simulink library "fast_library"  (Simulink 8.1)
settings: Solver=ode45  StartTime=0.0  StopTime=10.0  RelTol=1e-3
libraries: xbsIndex_r4 x439, casper_library_misc x3, xps_library x2
(part 2 of 3)

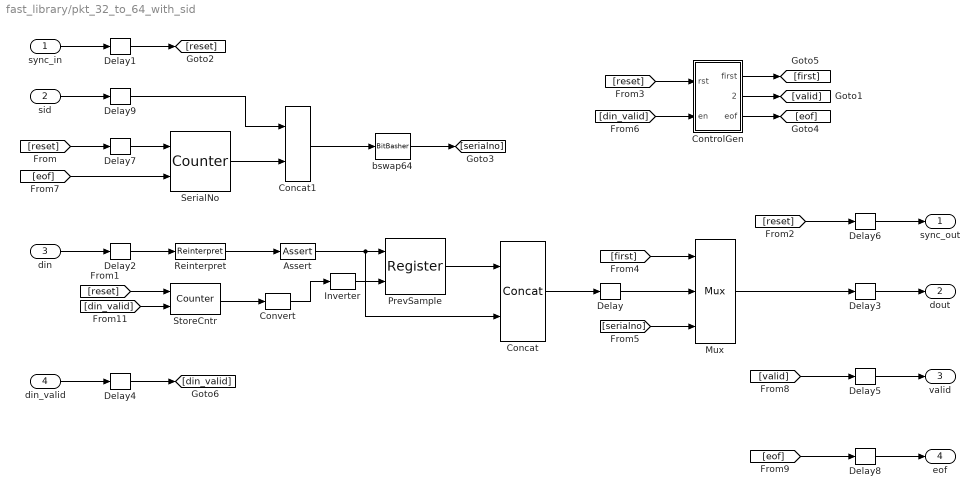
== system fast_library/pkt_32_to_64_with_sid ==
  sync_in : Inport
  sid : Inport  Port=2
  din : Inport  Port=3
  din_valid : Inport  Port=4
  Assert : xbsIndex_r4/Assert  assert_type=on  type_source=Explicitly  gui_display_data_type=Fixed-point  arith_type=Unsigned  n_bits=32  bin_pt=0  preci_type=Single  exp_width=8  frac_width=24  assert_rate=off  rate_source=Explicitly  period=1  output_port=on  block_type=assert
  Concat : xbsIndex_r4/Concat  num_inputs=2  dbl_ovrd=off  block_type=concat
  Concat1 : xbsIndex_r4/Concat  num_inputs=2  dbl_ovrd=off  block_type=concat
  ControlGen : Subsystem
  Convert : xbsIndex_r4/Convert  gui_display_data_type=Boolean  arith_type=Boolean  n_bits=16  bin_pt=14  float_type=Single  exp_bits=8  fraction_bits=24  quantization=Truncate  overflow=Wrap  en=off  latency=0  dbl_ovrd=off  pipeline=off  block_type=convert
  Delay{,1..5,7..9} (9 alike) : xbsIndex_r4/Delay  rst=off  infoeditControl=Selection of Reset will increase slice count due to use of real FFs and instead of SRLs  en=off  latency=1  dbl_ovrd=off  reg_retiming=off  block_type=delay
  Delay6 : xbsIndex_r4/Delay  rst=off  infoeditControl=Selection of Reset will increase slice count due to use of real FFs and instead of SRLs  en=off  latency=2  dbl_ovrd=off  reg_retiming=off  block_type=delay
  Inverter : xbsIndex_r4/Inverter  en=off  latency=0  dbl_ovrd=off  block_type=inv
  Mux : xbsIndex_r4/Mux  inputs=2  en=off  latency=0  precision=Full  arith_type=Unsigned  n_bits=16  bin_pt=14  quantization=Truncate  overflow=Wrap  dbl_ovrd=off  block_type=mux
  PrevSample : xbsIndex_r4/Register  init=0  rst=off  en=on  dbl_ovrd=off  block_type=register
  Reinterpret : xbsIndex_r4/Reinterpret  force_arith_type=on  arith_type=Unsigned  force_bin_pt=on  bin_pt=0  block_type=reinterpret
  SerialNo : xbsIndex_r4/Counter  cnt_type=Free Running  cnt_to=Inf  operation=Up  start_count=0  cnt_by_val=1  arith_type=Unsigned  n_bits=56  bin_pt=0  load_pin=off  rst=on  en=on  explicit_period=on  period=1  dbl_ovrd=off  use_behavioral_HDL=on  implementation=Fabric  block_type=counter
  StoreCntr : xbsIndex_r4/Counter  cnt_type=Free Running  cnt_to=Inf  operation=Up  start_count=0  cnt_by_val=1  arith_type=Unsigned  n_bits=1  bin_pt=0  load_pin=off  rst=on  en=on  explicit_period=on  period=1  dbl_ovrd=off  use_behavioral_HDL=off  implementation=Fabric  block_type=counter
  bswap64 : xbsIndex_r4/BitBasher  bitexpr=|  display_expr=off  sr_1=1  arith_type1=Unsigned  bin_pt1=0  sr_2=2  arith_type2=Unsigned  bin_pt2=0  sr_3=3  arith_type3=Unsigned  bin_pt3=0  sr_4=4  arith_type4=Unsigned  bin_pt4=0  dbl_ovrd=off  block_type=bitbasher
      | <!DOCTYPE HTML PUBLIC "-//W3C//DTD HTML 4.0//EN" "http://www.w3.org/TR/REC-html40/strict.dtd">
      | <html><head><meta name="qrichtext" content="1" /><style type="text/css">
      | p, li { white-space: pre-wrap; }
      | </style></head><body style=" font-family:'Segoe UI'; font-size:9pt; font-weight:400; font-style:normal;">
      | <p style=" margin-top:0px; margin-bottom:0px; margin-left:0px; margin-right:0px; -qt-block-indent:0; text-indent:0px;"><span style=" font-family:'MS Shell Dlg'; font-size:8pt;">b={a[7:0],a[15:8],a[23:16],a[31:24],a[39:32],a[47:40],a[55:48],a[63:56]}</span></p></body></html>
  sync_out : Outport
  dout : Outport  Port=2
  valid : Outport  Port=3
  eof : Outport  Port=4
  wires:
  ControlGen/3(eof) -> [eof]
  Convert/1 -> Inverter/1
  StoreCntr/1 -> Convert/1
  Inverter/1 -> PrevSample/2
  Concat/1 -> Delay/1
  [serialno] -> Mux/3
  PrevSample/1 -> Concat/1
  [reset] -> Delay7/1
  Delay/1 -> Mux/2
  din/1 -> Delay2/1
  [din_valid] -> ControlGen/2(en)
  [reset] -> ControlGen/1(rst)
  ControlGen/2(valid) -> [valid]
  sync_in/1 -> Delay1/1
  [reset] -> StoreCntr/1
  Reinterpret/1 -> Assert/1
  Assert/1 -> Concat/2, PrevSample/1
  Delay1/1 -> [reset]
  Delay2/1 -> Reinterpret/1
  Delay3/1 -> dout/1
  Mux/1 -> Delay3/1
  [reset] -> Delay6/1
  Delay6/1 -> sync_out/1
  [eof] -> SerialNo/2
  ControlGen/1(first) -> [first]
  [first] -> Mux/1
  Delay7/1 -> SerialNo/1
  din_valid/1 -> Delay4/1
  Delay4/1 -> [din_valid]
  [din_valid] -> StoreCntr/2
  Delay5/1 -> valid/1
  [valid] -> Delay5/1
  Delay8/1 -> eof/1
  [eof] -> Delay8/1
  bswap64/1 -> [serialno]
  sid/1 -> Delay9/1
  SerialNo/1 -> Concat1/2
  Delay9/1 -> Concat1/1
  Concat1/1 -> bswap64/1

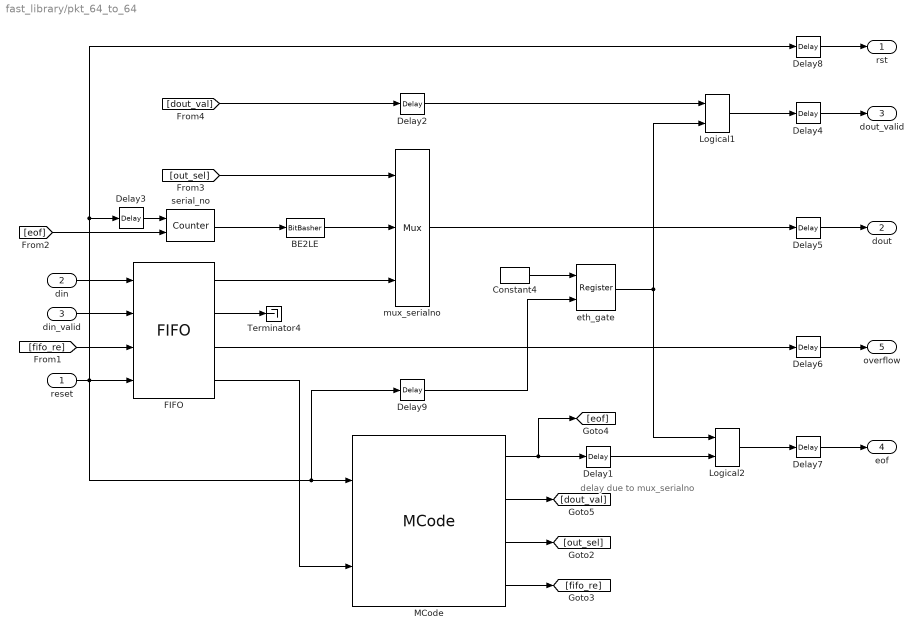
== system fast_library/pkt_64_to_64 ==
  note: delay due to mux_serialno
  reset : Inport
  din : Inport  Port=2
  din_valid : Inport  Port=3
  BE2LE : xbsIndex_r4/BitBasher  bitexpr=|  display_expr=off  sr_1=1  arith_type1=Unsigned  bin_pt1=0  sr_2=2  arith_type2=Unsigned  bin_pt2=0  sr_3=3  arith_type3=Unsigned  bin_pt3=0  sr_4=4  arith_type4=Unsigned  bin_pt4=0  dbl_ovrd=off  block_type=bitbasher
      | <!DOCTYPE HTML PUBLIC "-//W3C//DTD HTML 4.0//EN" "http://www.w3.org/TR/REC-html40/strict.dtd">
      | <html><head><meta name="qrichtext" content="1" /><style type="text/css">
      | p, li { white-space: pre-wrap; }
      | </style></head><body style=" font-family:'Segoe UI'; font-size:9pt; font-weight:400; font-style:normal;">
      | <p style=" margin-top:0px; margin-bottom:0px; margin-left:0px; margin-right:0px; -qt-block-indent:0; text-indent:0px;">out = {in[7:0], in[15:8], in[23:16], in[31:24], in[39:32], in[47:40], in[55:48], in[63:56]}</p></body></html>
  Constant4 : xbsIndex_r4/Constant  const=1  gui_display_data_type=Boolean  arith_type=Boolean  n_bits=11  bin_pt=0  preci_type=Single  exp_width=8  frac_width=24  explicit_period=on  period=1  equ=P=C  opselect=C  inp2=PCIN>>17  opr=+  inp1=P  carry=CIN  dbl_ovrd=off  block_type=constant
  Delay{1..2,4..7,9} (7 alike) : xbsIndex_r4/Delay  rst=off  infoeditControl=Selection of Reset will increase slice count due to use of real FFs and instead of SRLs  en=off  latency=2  dbl_ovrd=off  reg_retiming=off  block_type=delay
  Delay3 : xbsIndex_r4/Delay  rst=off  infoeditControl=Selection of Reset will increase slice count due to use of real FFs and instead of SRLs  en=off  latency=1  dbl_ovrd=off  reg_retiming=off  block_type=delay
  Delay8 : xbsIndex_r4/Delay  rst=off  infoeditControl=Selection of Reset will increase slice count due to use of real FFs and instead of SRLs  en=off  latency=1  dbl_ovrd=off  reg_retiming=off  block_type=delay
  FIFO : xbsIndex_r4/FIFO  mem_type=Block RAM  performance_options=Standard_FIFO  infoedit1=Available only for V4, V5, V6, V7, K7, A7 and Zynq devices.  embedded_registers=off  depth_sgadvanced=fifo_depth  depth=2K  percent_nbits=1  rst=on  en=off  use_dcount=on  use_percent_full_port=off  use_almost_empty=off  almost_empty_thresh=2  use_almost_full=off  almost_full_thresh=14  dbl_ovrd=off  explicit_period=off  block_type=fifo
      settings: has_advanced_control=1
  Logical1 : xbsIndex_r4/Logical  logical_function=AND  inputs=2  en=off  latency=0  precision=Full  arith_type=Unsigned  n_bits=16  bin_pt=0  align_bp=on  dbl_ovrd=off  block_type=logical
  Logical2 : xbsIndex_r4/Logical  logical_function=AND  inputs=2  en=off  latency=0  precision=Full  arith_type=Unsigned  n_bits=16  bin_pt=0  align_bp=on  dbl_ovrd=off  block_type=logical
  MCode : xbsIndex_r4/MCode  mfname=pktz_64to64_fsm  explicit_period=off  period=1  inputsTable={'boundInpExpr'=>['','','pktlen-1','pktlen-2','idlecycles-1'],'inputs'=>['reset','fifo_count','pktlen_m1','pktlen_m2','idlecycles_m1']}  outputsTable={'outputs'=>['eof','dval','out_sel','fifo_re'],'suppressOut'=>['off','off','off','off']}  dbl_ovrd=off  enable_stdout=off  enable_debug=off  suppress_output=on  defparams={'pktlen_m1',pktlen-1,'pktlen_m2',pktlen-2,'idlecycles_m1',idlecycles-1}  hide_port_list={}  block_type=mcode
  Terminator4 : Terminator
  eth_gate : xbsIndex_r4/Register  init=0  rst=off  en=on  dbl_ovrd=off  block_type=register
  mux_serialno : xbsIndex_r4/Mux  inputs=2  en=off  latency=2  precision=Full  arith_type=Unsigned  n_bits=16  bin_pt=14  quantization=Truncate  overflow=Wrap  dbl_ovrd=off  block_type=mux
  serial_no : xbsIndex_r4/Counter  cnt_type=Free Running  cnt_to=Inf  operation=Up  start_count=0  cnt_by_val=1  arith_type=Unsigned  n_bits=64  bin_pt=0  load_pin=off  rst=on  en=on  explicit_period=on  period=1  dbl_ovrd=off  use_behavioral_HDL=off  implementation=Fabric  block_type=counter
  rst : Outport
  dout : Outport  Port=2
  dout_valid : Outport  Port=3
  eof : Outport  Port=4
  overflow : Outport  Port=5
  wires:
  din_valid/1 -> FIFO/2
  din/1 -> FIFO/1
  reset/1 -> Delay8/1, Delay3/1, Delay9/1, MCode/1, FIFO/4
  Delay4/1 -> dout_valid/1
  Delay5/1 -> dout/1
  Delay6/1 -> overflow/1
  Delay7/1 -> eof/1
  [fifo_re] -> FIFO/3
  [eof] -> serial_no/2
  serial_no/1 -> BE2LE/1
  FIFO/1 -> mux_serialno/3
  [out_sel] -> mux_serialno/1
  MCode/2 -> [dout_val]
  mux_serialno/1 -> Delay5/1
  FIFO/3 -> Delay6/1
  [dout_val] -> Delay2/1
  MCode/1 -> [eof], Delay1/1
  MCode/3 -> [out_sel]
  MCode/4 -> [fifo_re]
  FIFO/4 -> MCode/2
  FIFO/2 -> Terminator4/1
  Delay3/1 -> serial_no/1
  BE2LE/1 -> mux_serialno/2
  Constant4/1 -> eth_gate/1
  Delay2/1 -> Logical1/1
  Logical1/1 -> Delay4/1
  eth_gate/1 -> Logical2/1, Logical1/2
  Delay1/1 -> Logical2/2
  Logical2/1 -> Delay7/1
  Delay8/1 -> rst/1
  Delay9/1 -> eth_gate/2

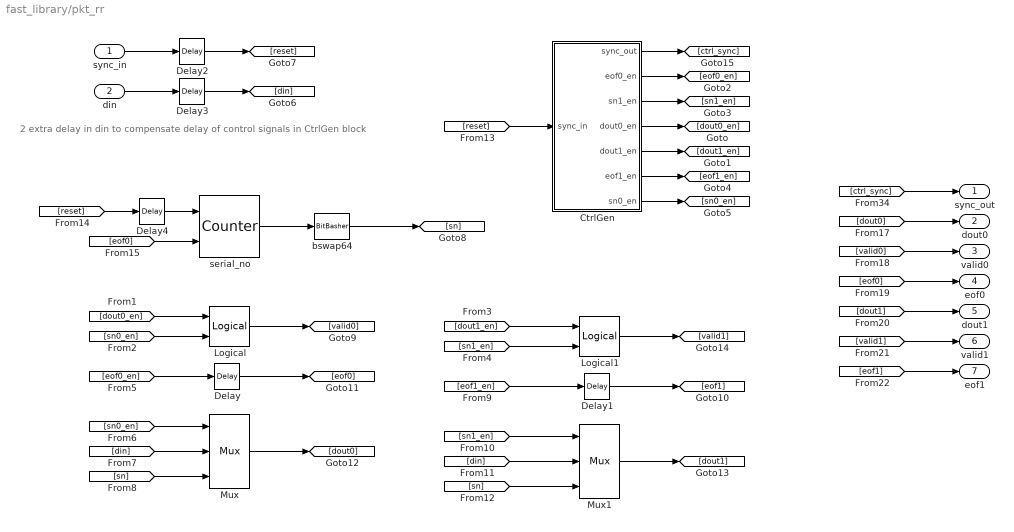
== system fast_library/pkt_rr ==
  note: 2 extra delay in din to compensate
      | delay of control signals in CtrlGen block
  sync_in : Inport
  din : Inport  Port=2
  CtrlGen : Subsystem  mask{nbits=nbits}
      mask prompts: nbits "Packet Size: (2^?)"
  Delay{,1..2,4} (4 alike) : xbsIndex_r4/Delay  rst=off  infoeditControl=Selection of Reset will increase slice count due to use of real FFs and instead of SRLs  en=off  latency=1  dbl_ovrd=off  reg_retiming=off  block_type=delay
  Delay3 : xbsIndex_r4/Delay  rst=off  infoeditControl=Selection of Reset will increase slice count due to use of real FFs and instead of SRLs  en=off  latency=3  dbl_ovrd=off  reg_retiming=off  block_type=delay
  Logical : xbsIndex_r4/Logical  logical_function=OR  inputs=2  en=off  latency=1  precision=Full  arith_type=Unsigned  n_bits=16  bin_pt=0  align_bp=on  dbl_ovrd=off  block_type=logical
  Logical1 : xbsIndex_r4/Logical  logical_function=OR  inputs=2  en=off  latency=1  precision=Full  arith_type=Unsigned  n_bits=16  bin_pt=0  align_bp=on  dbl_ovrd=off  block_type=logical
  Mux : xbsIndex_r4/Mux  inputs=2  en=off  latency=1  precision=Full  arith_type=Unsigned  n_bits=16  bin_pt=14  quantization=Truncate  overflow=Wrap  dbl_ovrd=off  block_type=mux
  Mux1 : xbsIndex_r4/Mux  inputs=2  en=off  latency=1  precision=Full  arith_type=Unsigned  n_bits=16  bin_pt=14  quantization=Truncate  overflow=Wrap  dbl_ovrd=off  block_type=mux
  bswap64 : xbsIndex_r4/BitBasher  bitexpr=|  display_expr=off  sr_1=1  arith_type1=Unsigned  bin_pt1=0  sr_2=2  arith_type2=Unsigned  bin_pt2=0  sr_3=3  arith_type3=Unsigned  bin_pt3=0  sr_4=4  arith_type4=Unsigned  bin_pt4=0  dbl_ovrd=off  block_type=bitbasher
      | <!DOCTYPE HTML PUBLIC "-//W3C//DTD HTML 4.0//EN" "http://www.w3.org/TR/REC-html40/strict.dtd">
      | <html><head><meta name="qrichtext" content="1" /><style type="text/css">
      | p, li { white-space: pre-wrap; }
      | </style></head><body style=" font-family:'Segoe UI'; font-size:9pt; font-weight:400; font-style:normal;">
      | <p style=" margin-top:12px; margin-bottom:12px; margin-left:0px; margin-right:0px; -qt-block-indent:0; text-indent:0px;"><span style=" font-family:'MS Shell Dlg'; font-size:8pt;">b={a[7:0],a[15:8],a[23:16],a[31:24],a[39:32],a[47:40],a[55:48],a[63:56]}</span></p></body></html>
  serial_no : xbsIndex_r4/Counter  cnt_type=Free Running  cnt_to=Inf  operation=Up  start_count=0  cnt_by_val=1  arith_type=Unsigned  n_bits=64  bin_pt=0  load_pin=off  rst=on  en=on  explicit_period=on  period=1  dbl_ovrd=off  use_behavioral_HDL=off  implementation=Fabric  block_type=counter
  sync_out : Outport
  dout0 : Outport  Port=2
  valid0 : Outport  Port=3
  eof0 : Outport  Port=4
  dout1 : Outport  Port=5
  valid1 : Outport  Port=6
  eof1 : Outport  Port=7
  wires:
  [dout0_en] -> Logical/1
  [sn0_en] -> Logical/2
  Logical/1 -> [valid0]
  [eof0_en] -> Delay/1
  Delay/1 -> [eof0]
  Mux/1 -> [dout0]
  [din] -> Mux/2
  [sn] -> Mux/3
  [dout1_en] -> Logical1/1
  [sn1_en] -> Logical1/2
  Logical1/1 -> [valid1]
  [eof1_en] -> Delay1/1
  Delay1/1 -> [eof1]
  Mux1/1 -> [dout1]
  [sn1_en] -> Mux1/1
  [din] -> Mux1/2
  [sn] -> Mux1/3
  [sn0_en] -> Mux/1
  CtrlGen/5(dout1_en) -> [dout1_en]
  CtrlGen/1(sync_out) -> [ctrl_sync]
  CtrlGen/4(dout0_en) -> [dout0_en]
  CtrlGen/2(eof0_en) -> [eof0_en]
  CtrlGen/7(sn0_en) -> [sn0_en]
  CtrlGen/6(eof1_en) -> [eof1_en]
  CtrlGen/3(sn1_en) -> [sn1_en]
  din/1 -> Delay3/1
  sync_in/1 -> Delay2/1
  [reset] -> CtrlGen/1(sync_in)
  [reset] -> Delay4/1
  Delay2/1 -> [reset]
  Delay3/1 -> [din]
  [eof0] -> serial_no/2
  serial_no/1 -> bswap64/1
  [dout0] -> dout0/1
  [valid0] -> valid0/1
  [eof0] -> eof0/1
  [dout1] -> dout1/1
  [valid1] -> valid1/1
  [eof1] -> eof1/1
  bswap64/1 -> [sn]
  [ctrl_sync] -> sync_out/1
  Delay4/1 -> serial_no/1

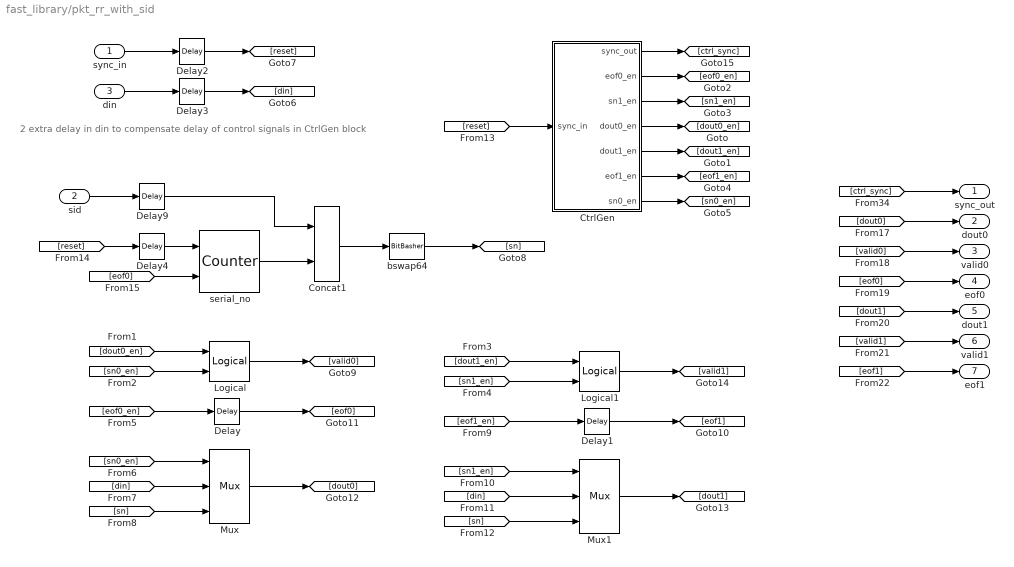
== system fast_library/pkt_rr_with_sid ==
  note: 2 extra delay in din to compensate
      | delay of control signals in CtrlGen block
  sync_in : Inport
  sid : Inport  Port=2
  din : Inport  Port=3
  Concat1 : xbsIndex_r4/Concat  num_inputs=2  dbl_ovrd=off  block_type=concat
  CtrlGen : Subsystem  mask{nbits=nbits}
      mask prompts: nbits "Packet Size: (2^?)"
  Delay{,1..2,4,9} (5 alike) : xbsIndex_r4/Delay  rst=off  infoeditControl=Selection of Reset will increase slice count due to use of real FFs and instead of SRLs  en=off  latency=1  dbl_ovrd=off  reg_retiming=off  block_type=delay
  Delay3 : xbsIndex_r4/Delay  rst=off  infoeditControl=Selection of Reset will increase slice count due to use of real FFs and instead of SRLs  en=off  latency=3  dbl_ovrd=off  reg_retiming=off  block_type=delay
  Logical : xbsIndex_r4/Logical  logical_function=OR  inputs=2  en=off  latency=1  precision=Full  arith_type=Unsigned  n_bits=16  bin_pt=0  align_bp=on  dbl_ovrd=off  block_type=logical
  Logical1 : xbsIndex_r4/Logical  logical_function=OR  inputs=2  en=off  latency=1  precision=Full  arith_type=Unsigned  n_bits=16  bin_pt=0  align_bp=on  dbl_ovrd=off  block_type=logical
  Mux : xbsIndex_r4/Mux  inputs=2  en=off  latency=1  precision=Full  arith_type=Unsigned  n_bits=16  bin_pt=14  quantization=Truncate  overflow=Wrap  dbl_ovrd=off  block_type=mux
  Mux1 : xbsIndex_r4/Mux  inputs=2  en=off  latency=1  precision=Full  arith_type=Unsigned  n_bits=16  bin_pt=14  quantization=Truncate  overflow=Wrap  dbl_ovrd=off  block_type=mux
  bswap64 : xbsIndex_r4/BitBasher  bitexpr=|  display_expr=off  sr_1=1  arith_type1=Unsigned  bin_pt1=0  sr_2=2  arith_type2=Unsigned  bin_pt2=0  sr_3=3  arith_type3=Unsigned  bin_pt3=0  sr_4=4  arith_type4=Unsigned  bin_pt4=0  dbl_ovrd=off  block_type=bitbasher
      | <!DOCTYPE HTML PUBLIC "-//W3C//DTD HTML 4.0//EN" "http://www.w3.org/TR/REC-html40/strict.dtd">
      | <html><head><meta name="qrichtext" content="1" /><style type="text/css">
      | p, li { white-space: pre-wrap; }
      | </style></head><body style=" font-family:'Segoe UI'; font-size:9pt; font-weight:400; font-style:normal;">
      | <p style=" margin-top:12px; margin-bottom:12px; margin-left:0px; margin-right:0px; -qt-block-indent:0; text-indent:0px;"><span style=" font-family:'MS Shell Dlg'; font-size:8pt;">b={a[7:0],a[15:8],a[23:16],a[31:24],a[39:32],a[47:40],a[55:48],a[63:56]}</span></p></body></html>
  serial_no : xbsIndex_r4/Counter  cnt_type=Free Running  cnt_to=Inf  operation=Up  start_count=0  cnt_by_val=1  arith_type=Unsigned  n_bits=64  bin_pt=0  load_pin=off  rst=on  en=on  explicit_period=on  period=1  dbl_ovrd=off  use_behavioral_HDL=off  implementation=Fabric  block_type=counter
  sync_out : Outport
  dout0 : Outport  Port=2
  valid0 : Outport  Port=3
  eof0 : Outport  Port=4
  dout1 : Outport  Port=5
  valid1 : Outport  Port=6
  eof1 : Outport  Port=7
  wires:
  Delay4/1 -> serial_no/1
  [ctrl_sync] -> sync_out/1
  bswap64/1 -> [sn]
  [eof1] -> eof1/1
  [valid1] -> valid1/1
  [dout1] -> dout1/1
  [eof0] -> eof0/1
  [valid0] -> valid0/1
  [dout0] -> dout0/1
  [eof0] -> serial_no/2
  Delay3/1 -> [din]
  Delay2/1 -> [reset]
  [reset] -> Delay4/1
  [reset] -> CtrlGen/1(sync_in)
  sync_in/1 -> Delay2/1
  din/1 -> Delay3/1
  CtrlGen/3(sn1_en) -> [sn1_en]
  CtrlGen/6(eof1_en) -> [eof1_en]
  CtrlGen/7(sn0_en) -> [sn0_en]
  CtrlGen/2(eof0_en) -> [eof0_en]
  CtrlGen/4(dout0_en) -> [dout0_en]
  CtrlGen/1(sync_out) -> [ctrl_sync]
  CtrlGen/5(dout1_en) -> [dout1_en]
  [sn0_en] -> Mux/1
  [sn] -> Mux1/3
  [din] -> Mux1/2
  [sn1_en] -> Mux1/1
  Mux1/1 -> [dout1]
  Delay1/1 -> [eof1]
  [eof1_en] -> Delay1/1
  Logical1/1 -> [valid1]
  [sn1_en] -> Logical1/2
  [dout1_en] -> Logical1/1
  [sn] -> Mux/3
  [din] -> Mux/2
  Mux/1 -> [dout0]
  Delay/1 -> [eof0]
  [eof0_en] -> Delay/1
  Logical/1 -> [valid0]
  [sn0_en] -> Logical/2
  [dout0_en] -> Logical/1
  sid/1 -> Delay9/1
  Delay9/1 -> Concat1/1
  serial_no/1 -> Concat1/2
  Concat1/1 -> bswap64/1

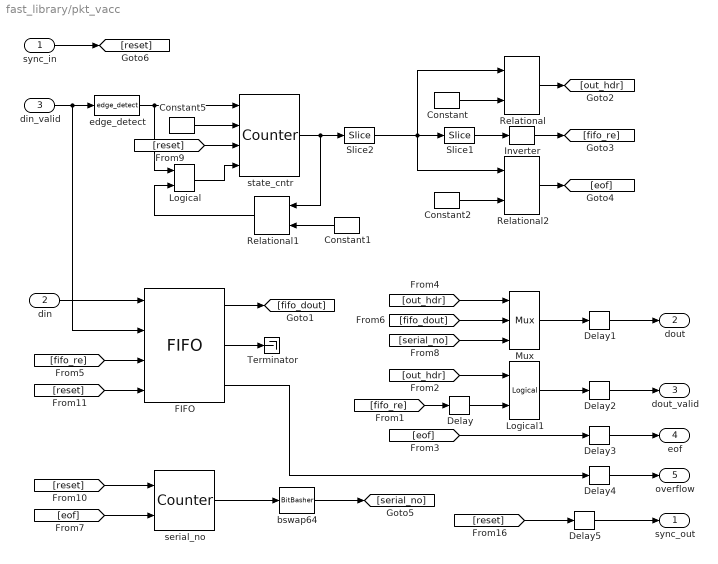
== system fast_library/pkt_vacc ==
  sync_in : Inport
  din : Inport  Port=2
  din_valid : Inport  Port=3
  Constant : xbsIndex_r4/Constant  const=0  gui_display_data_type=Fixed-point  arith_type=Unsigned  n_bits=pkt_bits+1  bin_pt=0  preci_type=Single  exp_width=8  frac_width=24  explicit_period=on  period=1  equ=P=C  opselect=C  inp2=PCIN>>17  opr=+  inp1=P  carry=CIN  dbl_ovrd=off  block_type=constant
  Constant1 : xbsIndex_r4/Constant  const=2^(spec_bits+1)-1  gui_display_data_type=Fixed-point  arith_type=Unsigned  n_bits=spec_bits+1  bin_pt=0  preci_type=Single  exp_width=8  frac_width=24  explicit_period=on  period=1  equ=P=C  opselect=C  inp2=PCIN>>17  opr=+  inp1=P  carry=CIN  dbl_ovrd=off  block_type=constant
  Constant2 : xbsIndex_r4/Constant  const=2^pkt_bits  gui_display_data_type=Fixed-point  arith_type=Unsigned  n_bits=pkt_bits+1  bin_pt=0  preci_type=Single  exp_width=8  frac_width=24  explicit_period=on  period=1  equ=P=C  opselect=C  inp2=PCIN>>17  opr=+  inp1=P  carry=CIN  dbl_ovrd=off  block_type=constant
  Constant5 : xbsIndex_r4/Constant  const=0  gui_display_data_type=Fixed-point  arith_type=Unsigned  n_bits=spec_bits+1  bin_pt=0  preci_type=Single  exp_width=8  frac_width=24  explicit_period=on  period=1  equ=P=C  opselect=C  inp2=PCIN>>17  opr=+  inp1=P  carry=CIN  dbl_ovrd=off  block_type=constant
  Delay{,1..4} (5 alike) : xbsIndex_r4/Delay  rst=off  infoeditControl=Selection of Reset will increase slice count due to use of real FFs and instead of SRLs  en=off  latency=1  dbl_ovrd=off  reg_retiming=off  block_type=delay
  Delay5 : xbsIndex_r4/Delay  rst=off  infoeditControl=Selection of Reset will increase slice count due to use of real FFs and instead of SRLs  en=off  latency=2  dbl_ovrd=off  reg_retiming=off  block_type=delay
  FIFO : xbsIndex_r4/FIFO  mem_type=Block RAM  performance_options=Standard_FIFO  infoedit1=Available only for V4, V5, V6, V7, K7, A7 and Zynq devices.  embedded_registers=off  depth_sgadvanced=fifo_depth  depth=16  percent_nbits=1  rst=on  en=off  use_dcount=off  use_percent_full_port=off  use_almost_empty=off  almost_empty_thresh=2  use_almost_full=off  almost_full_thresh=14  dbl_ovrd=off  explicit_period=off  block_type=fifo
      settings: has_advanced_control=1
  Inverter : xbsIndex_r4/Inverter  en=off  latency=0  dbl_ovrd=off  block_type=inv
  Logical : xbsIndex_r4/Logical  logical_function=OR  inputs=2  en=off  latency=0  precision=Full  arith_type=Unsigned  n_bits=16  bin_pt=0  align_bp=on  dbl_ovrd=off  block_type=logical
  Logical1 : xbsIndex_r4/Logical  logical_function=OR  inputs=2  en=off  latency=0  precision=Full  arith_type=Unsigned  n_bits=16  bin_pt=0  align_bp=on  dbl_ovrd=off  block_type=logical
  Mux : xbsIndex_r4/Mux  inputs=2  en=off  latency=0  precision=Full  arith_type=Unsigned  n_bits=16  bin_pt=14  quantization=Truncate  overflow=Wrap  dbl_ovrd=off  block_type=mux
  Relational : xbsIndex_r4/Relational  mode=a=b  en=off  latency=0  dbl_ovrd=off  block_type=relational
  Relational1 : xbsIndex_r4/Relational  mode=a!=b  en=off  latency=0  dbl_ovrd=off  block_type=relational
  Relational2 : xbsIndex_r4/Relational  mode=a=b  en=off  latency=0  dbl_ovrd=off  block_type=relational
  Slice1 : xbsIndex_r4/Slice  nbits=1  boolean_output=on  mode=Upper Bit Location + Width  bit1=0  base1=MSB of Input  bit0=0  base0=LSB of Input  dbl_ovrd=off  block_type=slice
  Slice2 : xbsIndex_r4/Slice  nbits=pkt_bits+1  boolean_output=off  mode=Lower Bit Location + Width  bit1=0  base1=MSB of Input  bit0=0  base0=LSB of Input  dbl_ovrd=off  block_type=slice
  Terminator : Terminator
  bswap64 : xbsIndex_r4/BitBasher  bitexpr=|  display_expr=off  sr_1=1  arith_type1=Unsigned  bin_pt1=0  sr_2=2  arith_type2=Unsigned  bin_pt2=0  sr_3=3  arith_type3=Unsigned  bin_pt3=0  sr_4=4  arith_type4=Unsigned  bin_pt4=0  dbl_ovrd=off  block_type=bitbasher
      | <!DOCTYPE HTML PUBLIC "-//W3C//DTD HTML 4.0//EN" "http://www.w3.org/TR/REC-html40/strict.dtd">
      | <html><head><meta name="qrichtext" content="1" /><style type="text/css">
      | p, li { white-space: pre-wrap; }
      | </style></head><body style=" font-family:'Segoe UI'; font-size:9pt; font-weight:400; font-style:normal;">
      | <p style=" margin-top:12px; margin-bottom:12px; margin-left:0px; margin-right:0px; -qt-block-indent:0; text-indent:0px;"><span style=" font-family:'MS Shell Dlg'; font-size:8pt;">b={a[7:0],a[15:8],a[23:16],a[31:24],a[39:32],a[47:40],a[55:48],a[63:56]}</span></p></body></html>
  edge_detect : casper_library_misc/edge_detect  edge=Rising  polarity=Active High  x_in=[0 0.08 0.08 0.16 0.16 0.24 0.24 0.32 0.32 0.4]  y_in="[-1 -1  1  1  1  1  1  1  1  1]"  x_out=[0.6 0.68 0.68 0.76 0.76 0.84 0.84 0.92 0.92 1]  y_out="[-1 -1  1  1 -1 -1 -1 -1 -1 -1]"
  serial_no : xbsIndex_r4/Counter  cnt_type=Free Running  cnt_to=Inf  operation=Up  start_count=0  cnt_by_val=1  arith_type=Unsigned  n_bits=64  bin_pt=0  load_pin=off  rst=on  en=on  explicit_period=on  period=1  dbl_ovrd=off  use_behavioral_HDL=on  implementation=Fabric  block_type=counter
  state_cntr : xbsIndex_r4/Counter  cnt_type=Free Running  cnt_to=2^8-1  operation=Up  start_count=2^(spec_bits+1)-1  cnt_by_val=1  arith_type=Unsigned  n_bits=spec_bits+1  bin_pt=0  load_pin=on  rst=on  en=on  explicit_period=on  period=1  dbl_ovrd=off  use_behavioral_HDL=on  implementation=Fabric  block_type=counter
  sync_out : Outport
  dout : Outport  Port=2
  dout_valid : Outport  Port=3
  eof : Outport  Port=4
  overflow : Outport  Port=5
  wires:
  Relational2/1 -> [eof]
  Constant2/1 -> Relational2/2
  Relational/1 -> [out_hdr]
  Inverter/1 -> [fifo_re]
  Constant/1 -> Relational/2
  [reset] -> FIFO/4
  Slice2/1 -> Relational2/1, Relational/1, Slice1/1
  [fifo_re] -> FIFO/3
  state_cntr/1 -> Relational1/1, Slice2/1
  Constant1/1 -> Relational1/2
  Constant5/1 -> state_cntr/2
  Logical/1 -> state_cntr/4
  edge_detect/1 -> state_cntr/1, Logical/1
  Relational1/1 -> Logical/2
  [reset] -> state_cntr/3
  din_valid/1 -> FIFO/2, edge_detect/1
  din/1 -> FIFO/1
  Slice1/1 -> Inverter/1
  FIFO/1 -> [fifo_dout]
  FIFO/2 -> Terminator/1
  FIFO/3 -> Delay4/1
  [fifo_re] -> Delay/1
  Delay/1 -> Logical1/2
  [out_hdr] -> Logical1/1
  Logical1/1 -> Delay2/1
  [eof] -> Delay3/1
  Mux/1 -> Delay1/1
  [out_hdr] -> Mux/1
  [fifo_dout] -> Mux/2
  serial_no/1 -> bswap64/1
  sync_in/1 -> [reset]
  [serial_no] -> Mux/3
  Delay1/1 -> dout/1
  Delay2/1 -> dout_valid/1
  Delay3/1 -> eof/1
  [eof] -> serial_no/2
  [reset] -> serial_no/1
  Delay4/1 -> overflow/1
  [reset] -> Delay5/1
  Delay5/1 -> sync_out/1
  bswap64/1 -> [serial_no]

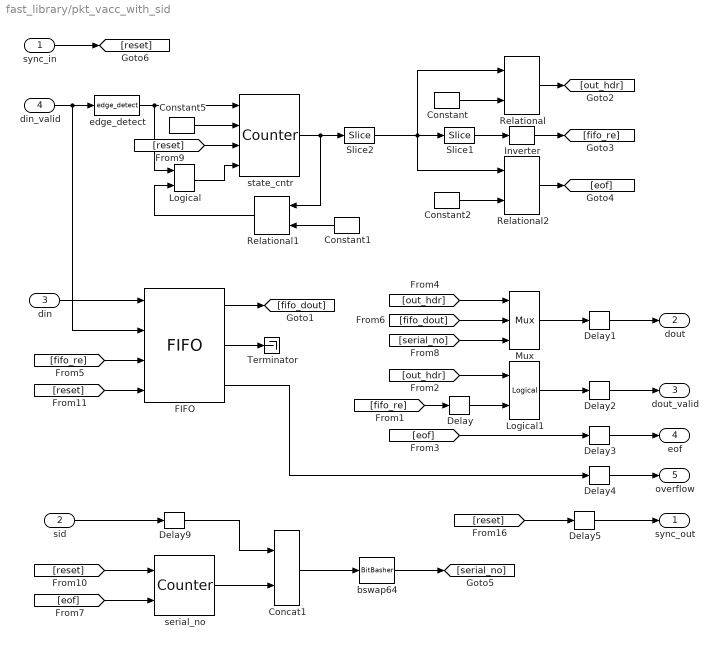
== system fast_library/pkt_vacc_with_sid ==
  sync_in : Inport
  sid : Inport  Port=2
  din : Inport  Port=3
  din_valid : Inport  Port=4
  Concat1 : xbsIndex_r4/Concat  num_inputs=2  dbl_ovrd=off  block_type=concat
  Constant : xbsIndex_r4/Constant  const=0  gui_display_data_type=Fixed-point  arith_type=Unsigned  n_bits=pkt_bits+1  bin_pt=0  preci_type=Single  exp_width=8  frac_width=24  explicit_period=on  period=1  equ=P=C  opselect=C  inp2=PCIN>>17  opr=+  inp1=P  carry=CIN  dbl_ovrd=off  block_type=constant
  Constant1 : xbsIndex_r4/Constant  const=2^(spec_bits+1)-1  gui_display_data_type=Fixed-point  arith_type=Unsigned  n_bits=spec_bits+1  bin_pt=0  preci_type=Single  exp_width=8  frac_width=24  explicit_period=on  period=1  equ=P=C  opselect=C  inp2=PCIN>>17  opr=+  inp1=P  carry=CIN  dbl_ovrd=off  block_type=constant
  Constant2 : xbsIndex_r4/Constant  const=2^pkt_bits  gui_display_data_type=Fixed-point  arith_type=Unsigned  n_bits=pkt_bits+1  bin_pt=0  preci_type=Single  exp_width=8  frac_width=24  explicit_period=on  period=1  equ=P=C  opselect=C  inp2=PCIN>>17  opr=+  inp1=P  carry=CIN  dbl_ovrd=off  block_type=constant
  Constant5 : xbsIndex_r4/Constant  const=0  gui_display_data_type=Fixed-point  arith_type=Unsigned  n_bits=spec_bits+1  bin_pt=0  preci_type=Single  exp_width=8  frac_width=24  explicit_period=on  period=1  equ=P=C  opselect=C  inp2=PCIN>>17  opr=+  inp1=P  carry=CIN  dbl_ovrd=off  block_type=constant
  Delay{,1..4,9} (6 alike) : xbsIndex_r4/Delay  rst=off  infoeditControl=Selection of Reset will increase slice count due to use of real FFs and instead of SRLs  en=off  latency=1  dbl_ovrd=off  reg_retiming=off  block_type=delay
  Delay5 : xbsIndex_r4/Delay  rst=off  infoeditControl=Selection of Reset will increase slice count due to use of real FFs and instead of SRLs  en=off  latency=2  dbl_ovrd=off  reg_retiming=off  block_type=delay
  FIFO : xbsIndex_r4/FIFO  mem_type=Block RAM  performance_options=Standard_FIFO  infoedit1=Available only for V4, V5, V6, V7, K7, A7 and Zynq devices.  embedded_registers=off  depth_sgadvanced=fifo_depth  depth=16  percent_nbits=1  rst=on  en=off  use_dcount=off  use_percent_full_port=off  use_almost_empty=off  almost_empty_thresh=2  use_almost_full=off  almost_full_thresh=14  dbl_ovrd=off  explicit_period=off  block_type=fifo
      settings: has_advanced_control=1
  Inverter : xbsIndex_r4/Inverter  en=off  latency=0  dbl_ovrd=off  block_type=inv
  Logical : xbsIndex_r4/Logical  logical_function=OR  inputs=2  en=off  latency=0  precision=Full  arith_type=Unsigned  n_bits=16  bin_pt=0  align_bp=on  dbl_ovrd=off  block_type=logical
  Logical1 : xbsIndex_r4/Logical  logical_function=OR  inputs=2  en=off  latency=0  precision=Full  arith_type=Unsigned  n_bits=16  bin_pt=0  align_bp=on  dbl_ovrd=off  block_type=logical
  Mux : xbsIndex_r4/Mux  inputs=2  en=off  latency=0  precision=Full  arith_type=Unsigned  n_bits=16  bin_pt=14  quantization=Truncate  overflow=Wrap  dbl_ovrd=off  block_type=mux
  Relational : xbsIndex_r4/Relational  mode=a=b  en=off  latency=0  dbl_ovrd=off  block_type=relational
  Relational1 : xbsIndex_r4/Relational  mode=a!=b  en=off  latency=0  dbl_ovrd=off  block_type=relational
  Relational2 : xbsIndex_r4/Relational  mode=a=b  en=off  latency=0  dbl_ovrd=off  block_type=relational
  Slice1 : xbsIndex_r4/Slice  nbits=1  boolean_output=on  mode=Upper Bit Location + Width  bit1=0  base1=MSB of Input  bit0=0  base0=LSB of Input  dbl_ovrd=off  block_type=slice
  Slice2 : xbsIndex_r4/Slice  nbits=pkt_bits+1  boolean_output=off  mode=Lower Bit Location + Width  bit1=0  base1=MSB of Input  bit0=0  base0=LSB of Input  dbl_ovrd=off  block_type=slice
  Terminator : Terminator
  bswap64 : xbsIndex_r4/BitBasher  bitexpr=|  display_expr=off  sr_1=1  arith_type1=Unsigned  bin_pt1=0  sr_2=2  arith_type2=Unsigned  bin_pt2=0  sr_3=3  arith_type3=Unsigned  bin_pt3=0  sr_4=4  arith_type4=Unsigned  bin_pt4=0  dbl_ovrd=off  block_type=bitbasher
      | <!DOCTYPE HTML PUBLIC "-//W3C//DTD HTML 4.0//EN" "http://www.w3.org/TR/REC-html40/strict.dtd">
      | <html><head><meta name="qrichtext" content="1" /><style type="text/css">
      | p, li { white-space: pre-wrap; }
      | </style></head><body style=" font-family:'Segoe UI'; font-size:9pt; font-weight:400; font-style:normal;">
      | <p style=" margin-top:12px; margin-bottom:12px; margin-left:0px; margin-right:0px; -qt-block-indent:0; text-indent:0px;"><span style=" font-family:'MS Shell Dlg'; font-size:8pt;">b={a[7:0],a[15:8],a[23:16],a[31:24],a[39:32],a[47:40],a[55:48],a[63:56]}</span></p></body></html>
  edge_detect : casper_library_misc/edge_detect  edge=Rising  polarity=Active High  x_in=[0 0.08 0.08 0.16 0.16 0.24 0.24 0.32 0.32 0.4]  y_in="[-1 -1  1  1  1  1  1  1  1  1]"  x_out=[0.6 0.68 0.68 0.76 0.76 0.84 0.84 0.92 0.92 1]  y_out="[-1 -1  1  1 -1 -1 -1 -1 -1 -1]"
  serial_no : xbsIndex_r4/Counter  cnt_type=Free Running  cnt_to=Inf  operation=Up  start_count=0  cnt_by_val=1  arith_type=Unsigned  n_bits=64  bin_pt=0  load_pin=off  rst=on  en=on  explicit_period=on  period=1  dbl_ovrd=off  use_behavioral_HDL=on  implementation=Fabric  block_type=counter
  state_cntr : xbsIndex_r4/Counter  cnt_type=Free Running  cnt_to=2^8-1  operation=Up  start_count=2^(spec_bits+1)-1  cnt_by_val=1  arith_type=Unsigned  n_bits=spec_bits+1  bin_pt=0  load_pin=on  rst=on  en=on  explicit_period=on  period=1  dbl_ovrd=off  use_behavioral_HDL=on  implementation=Fabric  block_type=counter
  sync_out : Outport
  dout : Outport  Port=2
  dout_valid : Outport  Port=3
  eof : Outport  Port=4
  overflow : Outport  Port=5
  wires:
  bswap64/1 -> [serial_no]
  Delay5/1 -> sync_out/1
  [reset] -> Delay5/1
  Delay4/1 -> overflow/1
  [reset] -> serial_no/1
  [eof] -> serial_no/2
  Delay3/1 -> eof/1
  Delay2/1 -> dout_valid/1
  Delay1/1 -> dout/1
  [serial_no] -> Mux/3
  sync_in/1 -> [reset]
  [fifo_dout] -> Mux/2
  [out_hdr] -> Mux/1
  Mux/1 -> Delay1/1
  [eof] -> Delay3/1
  Logical1/1 -> Delay2/1
  [out_hdr] -> Logical1/1
  Delay/1 -> Logical1/2
  [fifo_re] -> Delay/1
  FIFO/3 -> Delay4/1
  FIFO/2 -> Terminator/1
  FIFO/1 -> [fifo_dout]
  Slice1/1 -> Inverter/1
  din/1 -> FIFO/1
  din_valid/1 -> edge_detect/1, FIFO/2
  [reset] -> state_cntr/3
  Relational1/1 -> Logical/2
  edge_detect/1 -> Logical/1, state_cntr/1
  Logical/1 -> state_cntr/4
  Constant5/1 -> state_cntr/2
  Constant1/1 -> Relational1/2
  state_cntr/1 -> Slice2/1, Relational1/1
  [fifo_re] -> FIFO/3
  Slice2/1 -> Slice1/1, Relational/1, Relational2/1
  [reset] -> FIFO/4
  Constant/1 -> Relational/2
  Inverter/1 -> [fifo_re]
  Relational/1 -> [out_hdr]
  Constant2/1 -> Relational2/2
  Relational2/1 -> [eof]
  sid/1 -> Delay9/1
  serial_no/1 -> Concat1/2
  Delay9/1 -> Concat1/1
  Concat1/1 -> bswap64/1

== system fast_library/ppsarm ==
  note: Total Delay: 2 clocks
  reset : Inport
  PPS : Inport  Port=2
  ARM : Inport  Port=3
  Constant : xbsIndex_r4/Constant  const=1  gui_display_data_type=Boolean  arith_type=Boolean  n_bits=1  bin_pt=0  preci_type=Single  exp_width=8  frac_width=24  explicit_period=on  period=1  equ=P=C  opselect=C  inp2=PCIN>>17  opr=+  inp1=P  carry=CIN  dbl_ovrd=off  block_type=constant
  Delay{,1..3} (4 alike) : xbsIndex_r4/Delay  rst=off  infoeditControl=Selection of Reset will increase slice count due to use of real FFs and instead of SRLs  en=off  latency=1  dbl_ovrd=off  reg_retiming=off  block_type=delay
  Logical : xbsIndex_r4/Logical  logical_function=OR  inputs=2  en=off  latency=0  precision=Full  arith_type=Unsigned  n_bits=16  bin_pt=0  align_bp=on  dbl_ovrd=off  block_type=logical
  Logical1 : xbsIndex_r4/Logical  logical_function=AND  inputs=2  en=off  latency=0  precision=Full  arith_type=Unsigned  n_bits=16  bin_pt=0  align_bp=on  dbl_ovrd=off  block_type=logical
  Register : xbsIndex_r4/Register  init=0  rst=on  en=on  dbl_ovrd=off  block_type=register
  Slice : xbsIndex_r4/Slice  nbits=1  boolean_output=on  mode=Lower Bit Location + Width  bit1=0  base1=MSB of Input  bit0=0  base0=LSB of Input  dbl_ovrd=off  block_type=slice
  Slice1 : xbsIndex_r4/Slice  nbits=1  boolean_output=on  mode=Lower Bit Location + Width  bit1=0  base1=MSB of Input  bit0=0  base0=LSB of Input  dbl_ovrd=off  block_type=slice
  Slice2 : xbsIndex_r4/Slice  nbits=1  boolean_output=on  mode=Lower Bit Location + Width  bit1=0  base1=MSB of Input  bit0=0  base0=LSB of Input  dbl_ovrd=off  block_type=slice
  edge_detect : Subsystem  AncestorBlock=casper_library_misc/edge_detect  mask(edge_detect){edge=Rising, polarity=Active High, x_in=[0 0.08 0.08 0.16 0.16 0.24 0.24 0.32 0.32 0.4], y_in=[-1 -1  1  1  1  1  1  1  1  1], x_out=[0.6 0.68 0.68 0.76 0.76 0.84 0.84 0.92 0.92 1], y_out=[-1 -1  1  1 -1 -1 -1 -1 -1 -1]}
      mask prompts: edge "Edge Type"; polarity "Output Polarity"; x_in "Input X Positions"; y_in "Input Y Positions"; x_out "Output X Positions"; y_out "Output Y Positions"
      mask help: Output is active for one-cycle after each edge of the specified type (i.e. rising, falling or both).
      mask init: same as fast_library/noisecal/edge_detect1
      settings: AttributesFormatString=|
      | rising edges
      | active high
      mask Help: Output is active for one-cycle after each edge of the specified type (i.e. rising, falling, or both).  Latency is zero.
      mask TypeOptions edge: Rising | Falling | Both
      mask TypeOptions polarity: Active High | Active Low
      mask Display:
      | plot(x_in_num,0.5+y_in_num*0.2);
      | plot(x_out_num,0.5+y_out_num*0.2);
  edge_detect1 : Subsystem  AncestorBlock=casper_library_misc/edge_detect  mask(edge_detect){edge=Rising, polarity=Active High, x_in=[0 0.08 0.08 0.16 0.16 0.24 0.24 0.32 0.32 0.4], y_in=[-1 -1  1  1  1  1  1  1  1  1], x_out=[0.6 0.68 0.68 0.76 0.76 0.84 0.84 0.92 0.92 1], y_out=[-1 -1  1  1 -1 -1 -1 -1 -1 -1]}
      mask prompts: edge "Edge Type"; polarity "Output Polarity"; x_in "Input X Positions"; y_in "Input Y Positions"; x_out "Output X Positions"; y_out "Output Y Positions"
      mask help: Output is active for one-cycle after each edge of the specified type (i.e. rising, falling or both).
      mask init: same as fast_library/noisecal/edge_detect1
      settings: AttributesFormatString=|
      | rising edges
      | active high
      mask Help: Output is active for one-cycle after each edge of the specified type (i.e. rising, falling, or both).  Latency is zero.
      mask TypeOptions edge: Rising | Falling | Both
      mask TypeOptions polarity: Active High | Active Low
      mask Display:
      | plot(x_in_num,0.5+y_in_num*0.2);
      | plot(x_out_num,0.5+y_out_num*0.2);
  edge_detect2 : Subsystem  AncestorBlock=casper_library_misc/edge_detect  mask(edge_detect){edge=Rising, polarity=Active High, x_in=[0 0.08 0.08 0.16 0.16 0.24 0.24 0.32 0.32 0.4], y_in=[-1 -1  1  1  1  1  1  1  1  1], x_out=[0.6 0.68 0.68 0.76 0.76 0.84 0.84 0.92 0.92 1], y_out=[-1 -1  1  1 -1 -1 -1 -1 -1 -1]}
      mask prompts: edge "Edge Type"; polarity "Output Polarity"; x_in "Input X Positions"; y_in "Input Y Positions"; x_out "Output X Positions"; y_out "Output Y Positions"
      mask help: Output is active for one-cycle after each edge of the specified type (i.e. rising, falling or both).
      mask init: same as fast_library/noisecal/edge_detect1
      settings: AttributesFormatString=|
      | rising edges
      | active high
      mask Help: Output is active for one-cycle after each edge of the specified type (i.e. rising, falling, or both).  Latency is zero.
      mask TypeOptions edge: Rising | Falling | Both
      mask TypeOptions polarity: Active High | Active Low
      mask Display:
      | plot(x_in_num,0.5+y_in_num*0.2);
      | plot(x_out_num,0.5+y_out_num*0.2);
  PPSARMReset : Outport
  wires:
  Delay/1 -> edge_detect/1(in)
  Register/1 -> Logical1/2
  Delay2/1 -> edge_detect2/1(in)
  Delay1/1 -> edge_detect1/1(in)
  Delay3/1 -> PPSARMReset/1
  reset/1 -> Slice/1
  PPS/1 -> Slice1/1
  ARM/1 -> Slice2/1
  Logical1/1 -> Register/2, Logical/2
  edge_detect2/1(out) -> Register/3
  Slice/1 -> Delay/1
  Slice1/1 -> Delay1/1
  Slice2/1 -> Delay2/1
  Constant/1 -> Register/1
  edge_detect1/1(out) -> Logical1/1
  edge_detect/1(out) -> Logical/1
  Logical/1 -> Delay3/1

== system fast_library/pulse_ext ==
  in : Inport
  Constant : xbsIndex_r4/Constant  const=pulse_len  gui_display_data_type=Fixed-point  arith_type=Unsigned  n_bits=bits  bin_pt=0  preci_type=Single  exp_width=8  frac_width=24  explicit_period=on  period=1  equ=P=C  opselect=C  inp2=PCIN>>17  opr=+  inp1=P  carry=CIN  dbl_ovrd=off  block_type=constant
      settings: block_version=9.1.01
  Constant0 : xbsIndex_r4/Constant  const=0  gui_display_data_type=Fixed-point  arith_type=Unsigned  n_bits=bits  bin_pt=0  preci_type=Single  exp_width=8  frac_width=24  explicit_period=on  period=1  equ=P=C  opselect=C  inp2=PCIN>>17  opr=+  inp1=P  carry=CIN  dbl_ovrd=off  block_type=constant
      settings: block_version=9.1.01
  Counter : xbsIndex_r4/Counter  cnt_type=Free Running  cnt_to=1023  operation=Down  start_count=0  cnt_by_val=1  arith_type=Unsigned  n_bits=bits  bin_pt=0  load_pin=on  rst=off  en=on  explicit_period=on  period=1  dbl_ovrd=off  use_behavioral_HDL=off  implementation=Fabric  use_rpm=on  block_type=counter
      settings: xl_area=[0, 0, 0, 0, 0, 0, 0]  block_version=9.1.01
  Logical : xbsIndex_r4/Logical  logical_function=OR  inputs=2  en=off  latency=0  precision=Full  arith_type=Unsigned  n_bits=16  bin_pt=0  align_bp=on  dbl_ovrd=off  block_type=logical
  Relational : xbsIndex_r4/Relational  mode=a!=b  en=off  latency=0  dbl_ovrd=off  block_type=relational
      settings: xl_area=[0, 0, 0, 0, 0, 0, 0]  block_version=9.1.01
  posedge : Subsystem  Tag=Rising Edge Detector
  out : Outport
  wires:
  Logical/1 -> Counter/3
  Constant/1 -> Counter/2
  posedge/1(Out) -> Logical/1, Counter/1
  in/1 -> posedge/1(In)
  Relational/1 -> out/1, Logical/2
  Constant0/1 -> Relational/2
  Counter/1 -> Relational/1

== system fast_library/serial_to_parallel ==
  rst : Inport
  en : Inport  Port=2
  din : Inport  Port=3
  Concat : xbsIndex_r4/Concat  num_inputs=4  dbl_ovrd=off  block_type=concat
  Counter : xbsIndex_r4/Counter  cnt_type=Free Running  cnt_to=Inf  operation=Up  start_count=0  cnt_by_val=1  arith_type=Unsigned  n_bits=3  bin_pt=0  load_pin=on  rst=on  en=on  explicit_period=on  period=1  dbl_ovrd=off  use_behavioral_HDL=off  implementation=Fabric  block_type=counter
  Delay{,1..4} (5 alike) : xbsIndex_r4/Delay  rst=off  infoeditControl=Selection of Reset will increase slice count due to use of real FFs and instead of SRLs  en=off  latency=1  dbl_ovrd=off  reg_retiming=off  block_type=delay
  Expression : xbsIndex_r4/Expression  expression=(a&(~b))|c  align_bp=on  en=off  latency=0  precision=Full  arith_type=Unsigned  n_bits=16  bin_pt=0  dbl_ovrd=off  block_type=expr
  Logical : xbsIndex_r4/Logical  logical_function=AND  inputs=2  en=off  latency=0  precision=Full  arith_type=Unsigned  n_bits=16  bin_pt=0  align_bp=on  dbl_ovrd=off  block_type=logical
  Relational : xbsIndex_r4/Relational  mode=a=b  en=off  latency=0  dbl_ovrd=off  block_type=relational
  const_1 : xbsIndex_r4/Constant  const=1  gui_display_data_type=Fixed-point  arith_type=Unsigned  n_bits=3  bin_pt=0  preci_type=Single  exp_width=8  frac_width=24  explicit_period=on  period=1  equ=P=C  opselect=C  inp2=PCIN>>17  opr=+  inp1=P  carry=CIN  dbl_ovrd=off  block_type=constant
  en_buf : xbsIndex_r4/Delay  rst=off  infoeditControl=Selection of Reset will increase slice count due to use of real FFs and instead of SRLs  en=off  latency=1  dbl_ovrd=off  reg_retiming=off  block_type=delay
  num_elems : xbsIndex_r4/Constant  const=4  gui_display_data_type=Fixed-point  arith_type=Unsigned  n_bits=3  bin_pt=0  preci_type=Single  exp_width=8  frac_width=24  explicit_period=on  period=1  equ=P=C  opselect=C  inp2=PCIN>>17  opr=+  inp1=P  carry=CIN  dbl_ovrd=off  block_type=constant
  reg{1..4} (4 alike) : xbsIndex_r4/Register  init=0  rst=off  en=on  dbl_ovrd=off  block_type=register
  valid : Outport
  dout : Outport  Port=2
  wires:
  Counter/1 -> Relational/2
  num_elems/1 -> Relational/1
  reg1/1 -> Concat/1, reg2/1
  Logical/1 -> Counter/1
  Expression/1 -> Counter/3
  Relational/1 -> Expression/1, Logical/1, Delay2/1
  const_1/1 -> Counter/2
  en/1 -> en_buf/1, Delay/1
  din/1 -> Delay3/1
  rst/1 -> Delay1/1
  Delay/1 -> Counter/4, Logical/2, Expression/2
  Delay1/1 -> Expression/3
  Delay3/1 -> reg1/1
  en_buf/1 -> reg3/2, reg4/2, reg2/2, reg1/2
  Concat/1 -> Delay4/1
  reg2/1 -> Concat/2, reg3/1
  reg3/1 -> Concat/3, reg4/1
  Delay2/1 -> valid/1
  Delay4/1 -> dout/1
  reg4/1 -> Concat/4

== system fast_library/simple_qdr_vacc ==
  new_acc : Inport
  din : Inport  Port=2
  Adder : xbsIndex_r4/AddSub  mode=Addition  use_carryin=off  use_carryout=off  en=off  latency=2  precision=User Defined  arith_type="Signed  (2's comp)"  n_bits=n_bits  bin_pt=bin_pt  quantization=Truncate  overflow=Wrap  dbl_ovrd=off  use_behavioral_HDL=on  hw_selection=Fabric  pipelined=off  use_rpm=on  block_type=addsub
      settings: xl_area=[0, 0, 0, 0, 0, 0, 0]  block_version=10.1.3
  Constant : xbsIndex_r4/Constant  const=0  gui_display_data_type=Fixed-point  arith_type=Signed (2's comp)  n_bits=n_bits  bin_pt=bin_pt  preci_type=Single  exp_width=8  frac_width=24  explicit_period=on  period=1  equ=P=C  opselect=C  inp2=PCIN>>17  opr=+  inp1=P  carry=CIN  dbl_ovrd=off  block_type=constant
  Logical : xbsIndex_r4/Logical  logical_function=AND  inputs=2  en=off  latency=0  precision=Full  arith_type=Unsigned  n_bits=16  bin_pt=0  align_bp=on  dbl_ovrd=off  block_type=logical
  Mux2 : xbsIndex_r4/Mux  inputs=2  en=off  latency=0  precision=Full  arith_type="Signed  (2's comp)"  n_bits=8  bin_pt=2  quantization=Truncate  overflow=Wrap  dbl_ovrd=off  block_type=mux
      settings: xl_area=[0, 0, 0, 0, 0, 0, 0]
  Reinterpret : xbsIndex_r4/Reinterpret  force_arith_type=on  arith_type="Signed  (2's comp)"  force_bin_pt=on  bin_pt=bin_pt  block_type=reinterpret
  Slice : xbsIndex_r4/Slice  nbits=n_bits  boolean_output=off  mode=Lower Bit Location + Width  bit1=0  base1=MSB of Input  bit0=0  base0=LSB of Input  dbl_ovrd=off  block_type=slice
  delay_qdr : Subsystem  mask{DelayLen=vec_len-2, qdr_slot=qdr0}
      mask prompts: DelayLen "Delay Length (even number >=14):"; qdr_slot "QDR Slot:"
      mask init:
      | set_param([gcb, '/qdr'], 'which_qdr', qdr_slot);
      mask TypeOptions qdr_slot: qdr0 | qdr1 | qdr2 | qdr3
  pulse_ext1 : Subsystem  mask(pulse_ext){pulse_len=vec_len}
      mask prompts: pulse_len "Length of Pulse"
      mask help:
      | Extends a boolean signal to be high for the specified number of clocks after
      | the last high input.
      mask init:
      | bits = ceil(log2(pulse_len+1));
      mask Help: eval('xlWeb(''http://casper.berkeley.edu/wiki/Pulse_ext'')')
  dout : Outport
  valid : Outport  Port=2
  wires:
  new_acc/1 -> pulse_ext1/1(in)
  din/1 -> Adder/1
  Adder/1 -> delay_qdr/1(din)
  pulse_ext1/1(out) -> Logical/1, Mux2/1
  Mux2/1 -> Adder/2
  Constant/1 -> Mux2/3
  Logical/1 -> valid/1
  delay_qdr/2(valid) -> Logical/2
  Reinterpret/1 -> Mux2/2, dout/1
  Slice/1 -> Reinterpret/1
  delay_qdr/1(dout) -> Slice/1

== system fast_library/3-to-8 decoder/2-to-4 decoder ==
  A : Inport
  B : Inport  Port=2
  EN : Inport  Port=3
  Inverter : xbsIndex_r4/Inverter  en=off  latency=0  dbl_ovrd=off  block_type=inv
  Inverter1 : xbsIndex_r4/Inverter  en=off  latency=0  dbl_ovrd=off  block_type=inv
  Logical{,1..3} (4 alike) : xbsIndex_r4/Logical  logical_function=AND  inputs=3  en=off  latency=0  precision=Full  arith_type=Unsigned  n_bits=16  bin_pt=0  align_bp=on  dbl_ovrd=off  block_type=logical
  D0 : Outport
  D1 : Outport  Port=2
  D2 : Outport  Port=3
  D3 : Outport  Port=4
  wires:
  Logical2/1 -> D2/1
  Logical1/1 -> D1/1
  Logical/1 -> D0/1
  Inverter/1 -> Logical2/2, Logical/1
  B/1 -> Logical3/2, Logical2/1, Inverter1/1
  A/1 -> Logical3/1, Logical1/1, Inverter/1
  Logical3/1 -> D3/1
  Inverter1/1 -> Logical1/2, Logical/2
  EN/1 -> Logical1/3, Logical/3, Logical2/3, Logical3/3

== system fast_library/3-to-8 decoder/2-to-4 decoder1 ==
  A : Inport
  B : Inport  Port=2
  EN : Inport  Port=3
  Inverter : xbsIndex_r4/Inverter  en=off  latency=0  dbl_ovrd=off  block_type=inv
  Inverter1 : xbsIndex_r4/Inverter  en=off  latency=0  dbl_ovrd=off  block_type=inv
  Logical{,1..3} (4 alike) : xbsIndex_r4/Logical  logical_function=AND  inputs=3  en=off  latency=0  precision=Full  arith_type=Unsigned  n_bits=16  bin_pt=0  align_bp=on  dbl_ovrd=off  block_type=logical
  D0 : Outport
  D1 : Outport  Port=2
  D2 : Outport  Port=3
  D3 : Outport  Port=4
  wires:
  Logical2/1 -> D2/1
  Logical1/1 -> D1/1
  Logical/1 -> D0/1
  Inverter/1 -> Logical2/2, Logical/1
  B/1 -> Logical3/2, Logical2/1, Inverter1/1
  A/1 -> Logical3/1, Logical1/1, Inverter/1
  Logical3/1 -> D3/1
  Inverter1/1 -> Logical1/2, Logical/2
  EN/1 -> Logical1/3, Logical/3, Logical2/3, Logical3/3

== system fast_library/myrcs/id ==
  out_reg : Inport
  assert_reg : xbsIndex_r4/Assert  assert_type=on  type_source=Explicitly  gui_display_data_type=Fixed-point  arith_type=Unsigned  n_bits=32  bin_pt=0  preci_type=Single  exp_width=8  frac_width=24  assert_rate=off  rate_source=Explicitly  period=1  output_port=on  block_type=assert
  cast_gw : xbsIndex_r4/Convert  gui_display_data_type=Fixed-point  arith_type=Unsigned  n_bits=32  bin_pt=0  float_type=Single  exp_bits=8  fraction_bits=24  quantization=Truncate  overflow=Wrap  en=off  latency=0  dbl_ovrd=off  pipeline=off  block_type=convert
  io_delay : xbsIndex_r4/Delay  rst=off  infoeditControl=Selection of Reset will increase slice count due to use of real FFs and instead of SRLs  en=off  latency=0  dbl_ovrd=off  reg_retiming=on  block_type=delay
  myrcs_myrcs_id_user_data_in : xbsIndex_r4/Gateway Out  inherit_from_input=off  hdl_port=on  timing_constraint=None  locs_specified=off  LOCs={}  UseAsDAC=off  DACChannel='1'  block_type=gatewayout
  reint1 : xbsIndex_r4/Reinterpret  force_arith_type=on  arith_type=Unsigned  force_bin_pt=on  bin_pt=0  block_type=reinterpret
  sim_out : Terminator
  wires:
  reint1/1 -> io_delay/1
  assert_reg/1 -> reint1/1
  out_reg/1 -> assert_reg/1
  myrcs_myrcs_id_user_data_in/1 -> sim_out/1
  cast_gw/1 -> myrcs_myrcs_id_user_data_in/1
  io_delay/1 -> cast_gw/1

== system fast_library/myrcs/timestamp ==
  out_reg : Inport
  assert_reg : xbsIndex_r4/Assert  assert_type=on  type_source=Explicitly  gui_display_data_type=Fixed-point  arith_type=Unsigned  n_bits=32  bin_pt=0  preci_type=Single  exp_width=8  frac_width=24  assert_rate=off  rate_source=Explicitly  period=1  output_port=on  block_type=assert
  cast_gw : xbsIndex_r4/Convert  gui_display_data_type=Fixed-point  arith_type=Unsigned  n_bits=32  bin_pt=0  float_type=Single  exp_bits=8  fraction_bits=24  quantization=Truncate  overflow=Wrap  en=off  latency=0  dbl_ovrd=off  pipeline=off  block_type=convert
  io_delay : xbsIndex_r4/Delay  rst=off  infoeditControl=Selection of Reset will increase slice count due to use of real FFs and instead of SRLs  en=off  latency=0  dbl_ovrd=off  reg_retiming=on  block_type=delay
  myrcs_myrcs_timestamp_user_data_in : xbsIndex_r4/Gateway Out  inherit_from_input=off  hdl_port=on  timing_constraint=None  locs_specified=off  LOCs={}  UseAsDAC=off  DACChannel='1'  block_type=gatewayout
  reint1 : xbsIndex_r4/Reinterpret  force_arith_type=on  arith_type=Unsigned  force_bin_pt=on  bin_pt=0  block_type=reinterpret
  sim_out : Terminator
  wires:
  reint1/1 -> io_delay/1
  assert_reg/1 -> reint1/1
  out_reg/1 -> assert_reg/1
  myrcs_myrcs_timestamp_user_data_in/1 -> sim_out/1
  cast_gw/1 -> myrcs_myrcs_timestamp_user_data_in/1
  io_delay/1 -> cast_gw/1

== system fast_library/myrcs/ver ==
  out_reg : Inport
  assert_reg : xbsIndex_r4/Assert  assert_type=on  type_source=Explicitly  gui_display_data_type=Fixed-point  arith_type=Unsigned  n_bits=32  bin_pt=0  preci_type=Single  exp_width=8  frac_width=24  assert_rate=off  rate_source=Explicitly  period=1  output_port=on  block_type=assert
  cast_gw : xbsIndex_r4/Convert  gui_display_data_type=Fixed-point  arith_type=Unsigned  n_bits=32  bin_pt=0  float_type=Single  exp_bits=8  fraction_bits=24  quantization=Truncate  overflow=Wrap  en=off  latency=0  dbl_ovrd=off  pipeline=off  block_type=convert
  io_delay : xbsIndex_r4/Delay  rst=off  infoeditControl=Selection of Reset will increase slice count due to use of real FFs and instead of SRLs  en=off  latency=0  dbl_ovrd=off  reg_retiming=on  block_type=delay
  myrcs_myrcs_ver_user_data_in : xbsIndex_r4/Gateway Out  inherit_from_input=off  hdl_port=on  timing_constraint=None  locs_specified=off  LOCs={}  UseAsDAC=off  DACChannel='1'  block_type=gatewayout
  reint1 : xbsIndex_r4/Reinterpret  force_arith_type=on  arith_type=Unsigned  force_bin_pt=on  bin_pt=0  block_type=reinterpret
  sim_out : Terminator
  wires:
  reint1/1 -> io_delay/1
  assert_reg/1 -> reint1/1
  out_reg/1 -> assert_reg/1
  myrcs_myrcs_ver_user_data_in/1 -> sim_out/1
  cast_gw/1 -> myrcs_myrcs_ver_user_data_in/1
  io_delay/1 -> cast_gw/1
